simulink model "trasporto_impurezze"  (R2024b)
settings: Solver=VariableStepAuto  StartTime=0.0  StopTime=3  RelTol=1e-6
values from neighbouring files (symbols this model uses):
  ci_core = 2.05e19    (= 2.05e+19)    [fit_traporto_particelle.m]    (also in param_sparo_3.mat = 1.96393381569e+19)
  ci_omp = 1.0e19    (= 1e+19)    [fit_traporto_particelle.m]    (also in param_sparo_3.mat = 1.04458244578e+19)
  ci_T_core = 1071.06262207    [param_sparo_3.mat]
  ci_T_omp = 26.6552791595    [param_sparo_3.mat]
  ci_tar = 2.6e19    (= 2.6e+19)    [fit_traporto_particelle.m]    (also in param_sparo_3.mat = 1.50852693408e+19)
undefined symbols (not defined in the file or in its folder): ion, k0, Lz_valuesAzoto, V
libraries: slpidlib x3
settings Model: Creator=fedep  LastModifiedBy=costa

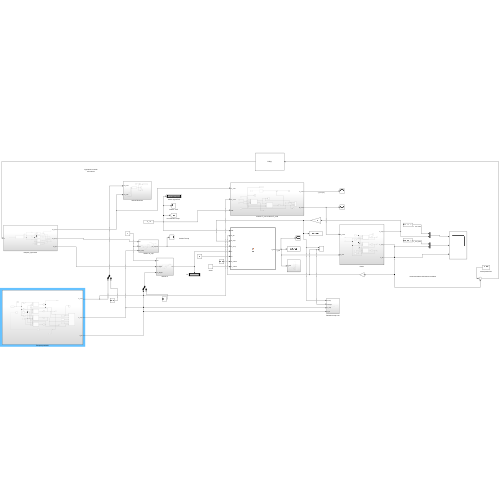
[thumbnail: Simulink's stored preview of the top-level diagram]
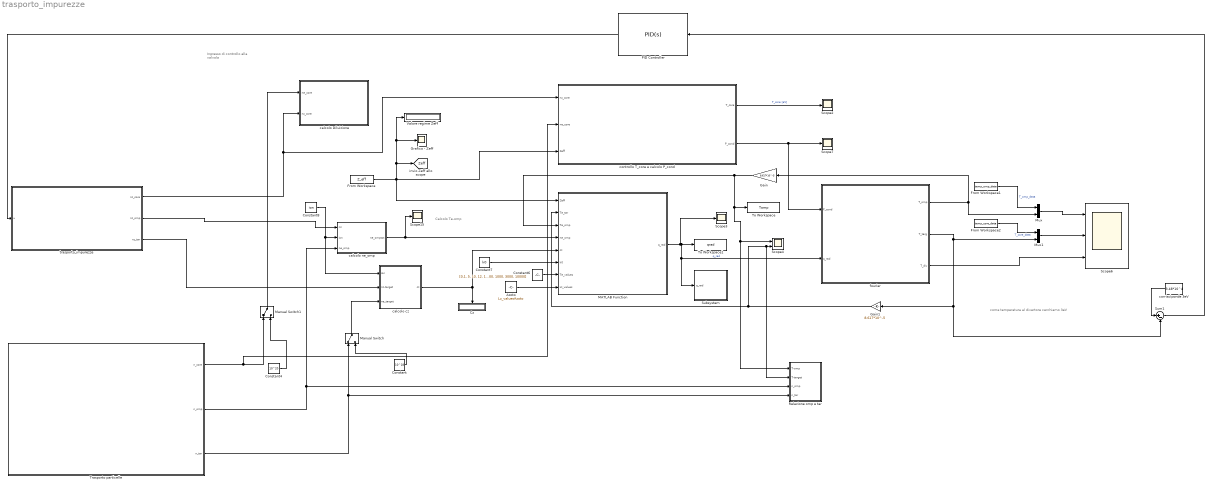
== system trasporto_impurezze ==
  note: come temperatura al divertore cerchiamo 3eV
  note: Ingresso di controllo
      | alla valvola
  note: Calcolo Te-omp
  Azoto : Constant  Value=Lz_valuesAzoto
  Constant : Constant  Value=10^18
  Constant4 : Constant  Value=10^20
  Constant6 : Constant  Value=[0,1, 5, 10, 12, 15, 20, 30, 59, 100, 155, 200, 300, 500, 700, 1000, 3000, 10000]
  Constant7 : Constant  Value=k0
  Constant8 : Constant  Value=ion
  Cz : Display
  From Workspace : FromWorkspace  VariableName=Z_eff
  From Workspace1 : FromWorkspace  VariableName=temp_omp_data
  From Workspace2 : FromWorkspace  VariableName=temp_core_data
  Gain : Gain  Gain=8.617*10^-5
  Gain1 : Gain  Gain=8.617*10^-5
  Grafico - Zeff : Scope
  MATLAB Function : MATLAB Function  TreatAsAtomicUnit=on
  Manual Switch : ManualSwitch
  Manual Switch1 : ManualSwitch
  Mux : Mux  Inputs=2
  Mux1 : Mux  Inputs=2
  PID Controller : slpidlib/PID Controller  Controller=PID  Form=Parallel  TimeDomain=Continuous-time  UseExternalTs=off  SampleTime=-1  IntegratorMethod=Forward Euler  FilterMethod=Forward Euler  ControllerParametersSource=internal  P=-7*10^9*0  I=-0.5*10^7*0  UseKiTs=off  D=-10^10*0  UseExternalDerivativeSource=off  N=100*0  UseFilter=on  TunerSelectOption=Transfer Function Based (PID Tuner App)  InitialConditionSource=internal  InitialConditionForIntegrator=0  InitialConditionForFilter=0  DifferentiatorICPrevScaledInput=0  ExternalReset=none  TrackingMode=off  Kt=1  LimitOutput=off  SatLimitsSource=internal  UpperSaturationLimit=inf  LowerSaturationLimit=-inf  LinearizeAsGain=on  AntiWindupMode=none  Kb=1  LimitIntegrator=off  UpperIntegratorSaturationLimit=inf  LowerIntegratorSaturationLimit=-inf  POutMin=[]  POutMax=[]  IOutMin=[]  IOutMax=[]  DOutMin=[]  DOutMax=[]  NOutMin=[]  NOutMax=[]  SumOutMin=[]  SumOutMax=[]  SaturationOutMin=[]  SaturationOutMax=[]  PParamMin=[]  PParamMax=[]  IParamMin=[]  IParamMax=[]  DParamMin=[]  DParamMax=[]  NParamMin=[]  NParamMax=[]  KbParamMin=[]  KbParamMax=[]  KtParamMin=[]  KtParamMax=[]  KbOutMin=[]  KbOutMax=[]  KtOutMin=[]  KtOutMax=[]  IntegratorOutMin=[]  IntegratorOutMax=[]  FilterOutMin=[]  FilterOutMax=[]  SumI1OutMin=[]  SumI1OutMax=[]  SumI2OutMin=[]  SumI2OutMax=[]  SumI3OutMin=[]  SumI3OutMax=[]  SumI4OutMin=[]  SumI4OutMax=[]  SumDOutMin=[]  SumDOutMax=[]  DifferentiatorOutMin=[]  DifferentiatorOutMax=[]  FilterDiffOutCoefMin=[]  FilterDiffOutCoefMax=[]  ReciprocalOutMin=[]  ReciprocalOutMax=[]  SumDenOutMin=[]  SumDenOutMax=[]  SumNumOutMin=[]  SumNumOutMax=[]  DivideOutMin=[]  DivideOutMax=[]  UdiffTsProdOutMin=[]  UdiffTsProdOutMax=[]  NTsProdOutMin=[]  NTsProdOutMax=[]  UintegralTsProdOutMin=[]  UintegralTsProdOutMax=[]  UngainTsProdOutMin=[]  UngainTsProdOutMax=[]  ClampingZeroOutDataTypeStr=Inherit: Inherit via back propagation  ClampingZeroOutMin=[]  ClampingZeroOutMax=[]  FilterDenConstantOutDataTypeStr=Inherit: Inherit via back propagation  FilterDenConstantOutMin=[]  FilterDenConstantOutMax=[]  PCopyOutDataTypeStr=Inherit: Inherit via back propagation  PCopyOutMin=[]  PCopyOutMax=[]  NCopyOutDataTypeStr=Inherit: Inherit via back propagation  NCopyOutMin=[]  NCopyOutMax=[]  IntegratorContinuousStateAttributes=''  IntegratorStateMustResolveToSignalObject=off  IntegratorRTWStateStorageClass=Auto  FilterContinuousStateAttributes=''  FilterStateMustResolveToSignalObject=off  FilterRTWStateStorageClass=Auto  ParallelPVariant=InternalParameters  IdealPVariant=Disabled  IVariant=InternalParameters  DVariant=InternalParameters  IntegratorVariant=Continuous  SatVariant=Disabled  AWVariant=Passthrough  PCopyVariant=Disabled  TRVariant=Disabled  FdbkBlocksVariant=Forward  IdealPFdbkVariant=Disabled  SatFdbkVariant=Disabled  DerivativeFilterVariant=ContFilter  NVariant=InternalParameters  NCopyVariant=Disabled  FilterICVariant=InternalICsFilter  IntegratorICVariant=InternalICs  ExternalResetVariant=Disabled  TRSumVariant=Passthrough  SumFdbkVariant=Disabled  SumVariant=Sum_PID  TsampFilterVariant=InternalTs  TsampNgainVariant=Passthrough  TsampIntegralVariant=Disabled_SignalSpec  ExternalSaturationOutDataTypeStr=Inherit: Same as second input  DerivativeSourceVariant=ErrorSignal  PreIntVariant=InternalPreInt
  Relazione omp e tar : Subsystem
  Scope{2..3,7,15} (4 alike) : Scope
  Scope4 : Scope  NumInputPorts=2
  Scope6 : Scope  NumInputPorts=3
  Subsystem : Subsystem
  Sum1 : Sum  Inputs=|+-
  To Workspace : ToWorkspace  VariableName=Tomp  SaveFormat=Timeseries  SampleTime=-1
  To Workspace1 : ToWorkspace  VariableName=qrad  SaveFormat=Timeseries  SampleTime=-1
  "Trasporto particelle " : Subsystem
  Valore regime Zeff : Display
  calcolo Diluizione : Subsystem
  calcolo cz : Subsystem
  calcolo ne_omp : Subsystem
  controllo T_core e calcolo P_cond : Subsystem
  corriscìponde 3eV : Constant  Value=3.48*10^4
  fourier : Subsystem
  trasporto_impurezze : Subsystem
  tag scope: Zeff=global
  wires:
  Constant6/1 -> MATLAB Function/7(Te_values)
  "Trasporto particelle "/1(n_core) -> controllo T_core e calcolo P_cond/2(ne_core), Manual Switch1/1
  "Trasporto particelle "/3(n_tar) -> Manual Switch/1, Relazione omp e tar/4(n_tar)
  Azoto/1 -> MATLAB Function/8(Lz_values)
  Manual Switch/1 -> calcolo cz/3(ne_target)
  Constant8/1 -> calcolo cz/1(ion), calcolo ne_omp/2(ion)
  From Workspace/1 -> controllo T_core e calcolo P_cond/3(Zeff), [Zeff], Grafico - Zeff/1, Valore regime Zeff/1, MATLAB Function/1(Zeff)
  Manual Switch1/1 -> calcolo Diluizione/1(ne_core)
  MATLAB Function/1(q_rad) -> To Workspace1/1, fourier/2(q_rad), Subsystem/1(q_rad), Scope3/1  "q_rad"
  "Trasporto particelle "/2(n_omp) -> calcolo ne_omp/3(ne_omp), Relazione omp e tar/3(n_omp)
  fourier/1(T_omp) -> Mux/2, Gain/1
  trasporto_impurezze/2(nz_omp) -> calcolo ne_omp/1(nz)
  PID Controller/1 -> trasporto_impurezze/1(u)
  fourier/3(T_div) -> Scope6/3
  Constant4/1 -> Manual Switch1/2
  corriscìponde 3eV/1 -> Sum1/1
  Sum1/1 -> PID Controller/1
  controllo T_core e calcolo P_cond/1(T_core) -> Scope2/1  "T_core [eV]"
  controllo T_core e calcolo P_cond/2(P_cond) -> Scope7/1, fourier/1(P_cond)
  calcolo ne_omp/1(ne_omptot) -> MATLAB Function/4(ne_omp), Scope15/1
  Gain/1 -> To Workspace/1, Relazione omp e tar/1(T-omp), Scope4/1, MATLAB Function/3(Te_omp)
  Constant/1 -> Manual Switch/2
  Constant7/1 -> MATLAB Function/6(k0)
  fourier/2(T_targ) -> Sum1/2, Gain1/1, Mux1/2
  Gain1/1 -> Scope4/2, Relazione omp e tar/2(T-target), MATLAB Function/2(Te_tar)
  calcolo cz/1(cz) -> Cz/1, MATLAB Function/5(cz)
  trasporto_impurezze/1(nz_core) -> calcolo Diluizione/2(nz_core), controllo T_core e calcolo P_cond/1(nz_core)
  trasporto_impurezze/3(nz_tar) -> calcolo cz/2(nz-target)
  From Workspace1/1 -> Mux/1  "T_omp_data"
  From Workspace2/1 -> Mux1/1  "T_core_data"
  Mux/1 -> Scope6/1
  Mux1/1 -> Scope6/2

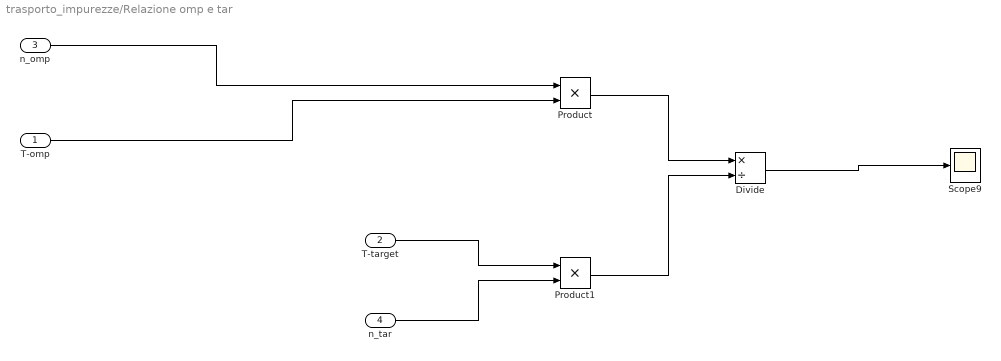
== system trasporto_impurezze/Relazione omp e tar ==
  T-omp : Inport
  T-target : Inport  Port=2
  n_omp : Inport  Port=3
  n_tar : Inport  Port=4
  Divide : Product  Inputs=*/
  Product : Product
  Product1 : Product
  Scope9 : Scope
  wires:
  Product/1 -> Divide/1
  n_tar/1 -> Product1/2
  Divide/1 -> Scope9/1
  Product1/1 -> Divide/2
  n_omp/1 -> Product/1
  T-target/1 -> Product1/1
  T-omp/1 -> Product/2

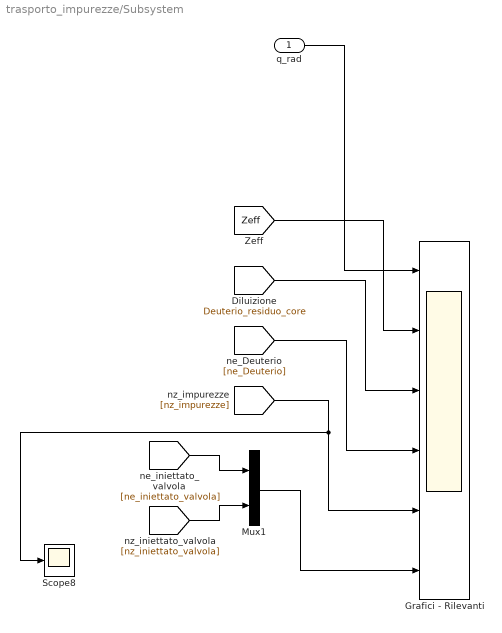
== system trasporto_impurezze/Subsystem ==
  q_rad : Inport
  Grafici - Rilevanti : Scope  NumInputPorts=6
  Mux1 : Mux  Inputs=2
  Scope8 : Scope
  wires:
  q_rad/1 -> Grafici - Rilevanti/1
  [Zeff] -> Grafici - Rilevanti/2
  [nz_impurezze] -> Scope8/1, Grafici - Rilevanti/5
  Mux1/1 -> Grafici - Rilevanti/6
  [nz_iniettato_valvola] -> Mux1/2
  [Deuterio_residuo_core] -> Grafici - Rilevanti/3
  [ne_Deuterio] -> Grafici - Rilevanti/4
  [ne_iniettato_valvola] -> Mux1/1

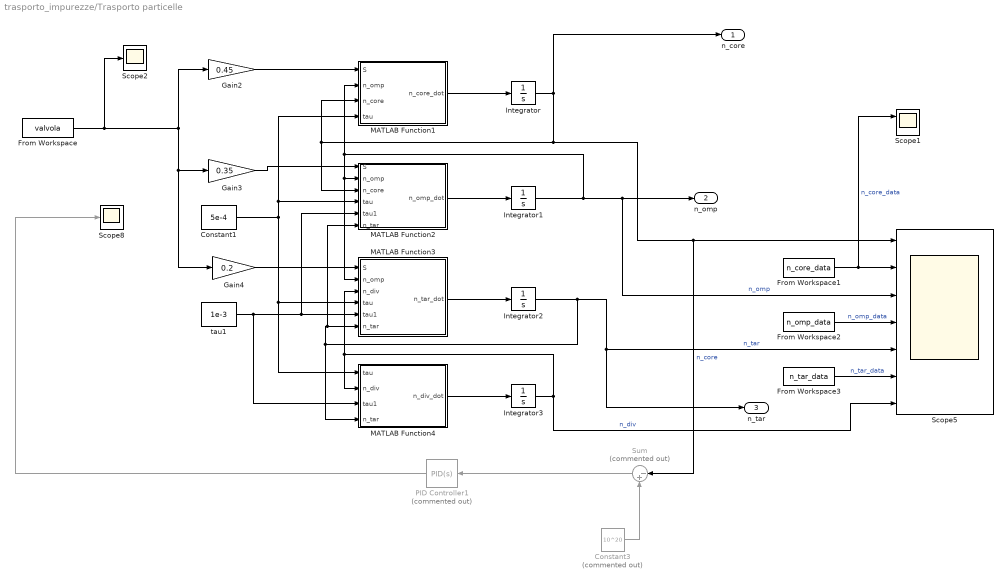
== system trasporto_impurezze/Trasporto particelle  ==
  Constant1 : Constant  Value=5e-4
  Constant3 : Constant  Commented=on  Value=10^20
  From Workspace : FromWorkspace  VariableName=valvola
  From Workspace1 : FromWorkspace  VariableName=n_core_data
  From Workspace2 : FromWorkspace  VariableName=n_omp_data
  From Workspace3 : FromWorkspace  VariableName=n_tar_data
  Gain2 : Gain  Gain=0.45
  Gain3 : Gain  Gain=0.35
  Gain4 : Gain  Gain=0.2
  Integrator : Integrator  InitialCondition=ci_core
  Integrator1 : Integrator  InitialCondition=ci_omp
  Integrator2 : Integrator  InitialCondition=ci_tar
  Integrator3 : Integrator  InitialCondition=10^10
  MATLAB Function1 : MATLAB Function  TreatAsAtomicUnit=on
  MATLAB Function2 : MATLAB Function  TreatAsAtomicUnit=on
  MATLAB Function3 : MATLAB Function  TreatAsAtomicUnit=on
  MATLAB Function4 : MATLAB Function  TreatAsAtomicUnit=on
  PID Controller1 : slpidlib/PID Controller  Commented=on  Controller=PID  Form=Parallel  TimeDomain=Continuous-time  UseExternalTs=off  SampleTime=-1  IntegratorMethod=Forward Euler  FilterMethod=Forward Euler  ControllerParametersSource=internal  P=10^2  I=0  UseKiTs=off  D=0  UseExternalDerivativeSource=off  N=100  UseFilter=on  TunerSelectOption=Transfer Function Based (PID Tuner App)  InitialConditionSource=internal  InitialConditionForIntegrator=0  InitialConditionForFilter=0  DifferentiatorICPrevScaledInput=0  ExternalReset=none  TrackingMode=off  Kt=1  LimitOutput=off  SatLimitsSource=internal  UpperSaturationLimit=inf  LowerSaturationLimit=-inf  LinearizeAsGain=on  AntiWindupMode=none  Kb=1  LimitIntegrator=off  UpperIntegratorSaturationLimit=inf  LowerIntegratorSaturationLimit=-inf  POutMin=[]  POutMax=[]  IOutMin=[]  IOutMax=[]  DOutMin=[]  DOutMax=[]  NOutMin=[]  NOutMax=[]  SumOutMin=[]  SumOutMax=[]  SaturationOutMin=[]  SaturationOutMax=[]  PParamMin=[]  PParamMax=[]  IParamMin=[]  IParamMax=[]  DParamMin=[]  DParamMax=[]  NParamMin=[]  NParamMax=[]  KbParamMin=[]  KbParamMax=[]  KtParamMin=[]  KtParamMax=[]  KbOutMin=[]  KbOutMax=[]  KtOutMin=[]  KtOutMax=[]  IntegratorOutMin=[]  IntegratorOutMax=[]  FilterOutMin=[]  FilterOutMax=[]  SumI1OutMin=[]  SumI1OutMax=[]  SumI2OutMin=[]  SumI2OutMax=[]  SumI3OutMin=[]  SumI3OutMax=[]  SumI4OutMin=[]  SumI4OutMax=[]  SumDOutMin=[]  SumDOutMax=[]  DifferentiatorOutMin=[]  DifferentiatorOutMax=[]  FilterDiffOutCoefMin=[]  FilterDiffOutCoefMax=[]  ReciprocalOutMin=[]  ReciprocalOutMax=[]  SumDenOutMin=[]  SumDenOutMax=[]  SumNumOutMin=[]  SumNumOutMax=[]  DivideOutMin=[]  DivideOutMax=[]  UdiffTsProdOutMin=[]  UdiffTsProdOutMax=[]  NTsProdOutMin=[]  NTsProdOutMax=[]  UintegralTsProdOutMin=[]  UintegralTsProdOutMax=[]  UngainTsProdOutMin=[]  UngainTsProdOutMax=[]  ClampingZeroOutDataTypeStr=Inherit: Inherit via back propagation  ClampingZeroOutMin=[]  ClampingZeroOutMax=[]  FilterDenConstantOutDataTypeStr=Inherit: Inherit via back propagation  FilterDenConstantOutMin=[]  FilterDenConstantOutMax=[]  PCopyOutDataTypeStr=Inherit: Inherit via back propagation  PCopyOutMin=[]  PCopyOutMax=[]  NCopyOutDataTypeStr=Inherit: Inherit via back propagation  NCopyOutMin=[]  NCopyOutMax=[]  IntegratorContinuousStateAttributes=''  IntegratorStateMustResolveToSignalObject=off  IntegratorRTWStateStorageClass=Auto  FilterContinuousStateAttributes=''  FilterStateMustResolveToSignalObject=off  FilterRTWStateStorageClass=Auto  ParallelPVariant=InternalParameters  IdealPVariant=Disabled  IVariant=InternalParameters  DVariant=InternalParameters  IntegratorVariant=Continuous  SatVariant=Disabled  AWVariant=Passthrough  PCopyVariant=Disabled  TRVariant=Disabled  FdbkBlocksVariant=Forward  IdealPFdbkVariant=Disabled  SatFdbkVariant=Disabled  DerivativeFilterVariant=ContFilter  NVariant=InternalParameters  NCopyVariant=Disabled  FilterICVariant=InternalICsFilter  IntegratorICVariant=InternalICs  ExternalResetVariant=Disabled  TRSumVariant=Passthrough  SumFdbkVariant=Disabled  SumVariant=Sum_PID  TsampFilterVariant=InternalTs  TsampNgainVariant=Passthrough  TsampIntegralVariant=Disabled_SignalSpec  ExternalSaturationOutDataTypeStr=Inherit: Same as second input  DerivativeSourceVariant=ErrorSignal  PreIntVariant=InternalPreInt
  Scope1 : Scope  NumInputPorts=2
  Scope2 : Scope
  Scope5 : Scope  NumInputPorts=7
  Scope8 : Scope
  Sum : Sum  Commented=on  Inputs=|-+
  tau1 : Constant  Value=1e-3
  n_core : Outport
  n_omp : Outport  Port=2
  n_tar : Outport  Port=3
  wires:
  Gain3/1 -> MATLAB Function2/1(S)
  Integrator2/1 -> n_tar/1, Scope5/5, MATLAB Function4/4(n_tar), MATLAB Function2/6(n_tar), MATLAB Function3/6(n_tar)  "n_tar"
  MATLAB Function2/1(n_omp_dot) -> Integrator1/1
  Integrator/1 -> n_core/1, Sum/1, Scope5/1, MATLAB Function1/3(n_core), MATLAB Function2/3(n_core)  "n_core"
  Integrator1/1 -> MATLAB Function3/2(n_omp), MATLAB Function2/2(n_omp), MATLAB Function1/2(n_omp), Scope5/3, n_omp/1  "n_omp"
  Constant1/1 -> MATLAB Function1/4(tau), MATLAB Function2/4(tau), MATLAB Function4/1(tau), MATLAB Function3/4(tau)
  Gain4/1 -> MATLAB Function3/1(S)
  Gain2/1 -> MATLAB Function1/1(S)
  MATLAB Function1/1(n_core_dot) -> Integrator/1
  Integrator3/1 -> MATLAB Function4/2(n_div), MATLAB Function3/3(n_div), Scope5/7  "n_div"
  MATLAB Function4/1(n_div_dot) -> Integrator3/1
  MATLAB Function3/1(n_tar_dot) -> Integrator2/1
  Sum/1 -> PID Controller1/1
  Constant3/1 -> Sum/2
  PID Controller1/1 -> Scope8/1
  From Workspace/1 -> Scope2/1, Gain2/1, Gain4/1, Gain3/1
  From Workspace1/1 -> Scope1/1, Scope5/2  "n_core_data"
  From Workspace2/1 -> Scope5/4  "n_omp_data"
  From Workspace3/1 -> Scope5/6  "n_tar_data"
  tau1/1 -> MATLAB Function4/3(tau1), MATLAB Function2/5(tau1), MATLAB Function3/5(tau1)

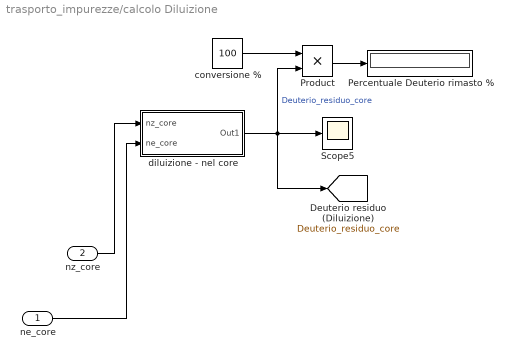
== system trasporto_impurezze/calcolo Diluizione ==
  ne_core : Inport
  nz_core : Inport  Port=2
  Percentuale Deuterio rimasto % : Display
  Product : Product
  Scope5 : Scope
  "conversione % " : Constant  Value=100
  diluizione - nel core : Subsystem
  tag scope: Deuterio_residuo_core=global
  wires:
  Product/1 -> Percentuale Deuterio rimasto %/1
  nz_core/1 -> diluizione - nel core/1(nz_core)
  "conversione % "/1 -> Product/1
  diluizione - nel core/1(Out1) -> [Deuterio_residuo_core], Scope5/1, Product/2  "Deuterio_residuo_core"
  ne_core/1 -> diluizione - nel core/2(ne_core)

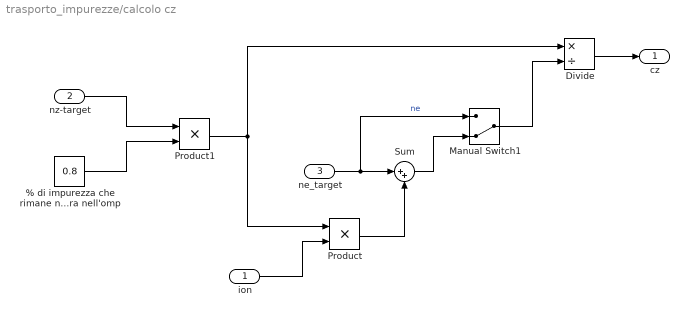
== system trasporto_impurezze/calcolo cz ==
  ion : Inport
  nz-target : Inport  Port=2
  ne_target : Inport  Port=3
  % di impurezza che rimane nel div. Parte restante migra nell'omp : Constant  Value=0.8
  Divide : Product  Inputs=*/
  Manual Switch1 : ManualSwitch  CurrentSetting=0
  Product : Product
  Product1 : Product
  Sum : Sum  Inputs=|++
  cz : Outport
  wires:
  ne_target/1 -> Manual Switch1/1, Sum/1  "ne"
  Sum/1 -> Manual Switch1/2
  Divide/1 -> cz/1
  Manual Switch1/1 -> Divide/2
  Product/1 -> Sum/2
  nz-target/1 -> Product1/1
  % di impurezza che rimane nel div. Parte restante migra nell'omp/1 -> Product1/2
  ion/1 -> Product/2
  Product1/1 -> Divide/1, Product/1

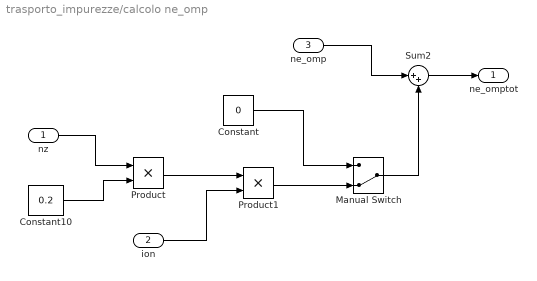
== system trasporto_impurezze/calcolo ne_omp ==
  nz : Inport
  ion : Inport  Port=2
  ne_omp : Inport  Port=3
  Constant : Constant  Value=0
  Constant10 : Constant  Value=0.2
  Manual Switch : ManualSwitch  CurrentSetting=0
  Product : Product
  Product1 : Product
  Sum2 : Sum  Inputs=|++
  ne_omptot : Outport
  wires:
  Constant10/1 -> Product/2
  Sum2/1 -> ne_omptot/1
  nz/1 -> Product/1
  ne_omp/1 -> Sum2/1
  Constant/1 -> Manual Switch/1
  Manual Switch/1 -> Sum2/2
  Product/1 -> Product1/1
  ion/1 -> Product1/2
  Product1/1 -> Manual Switch/2

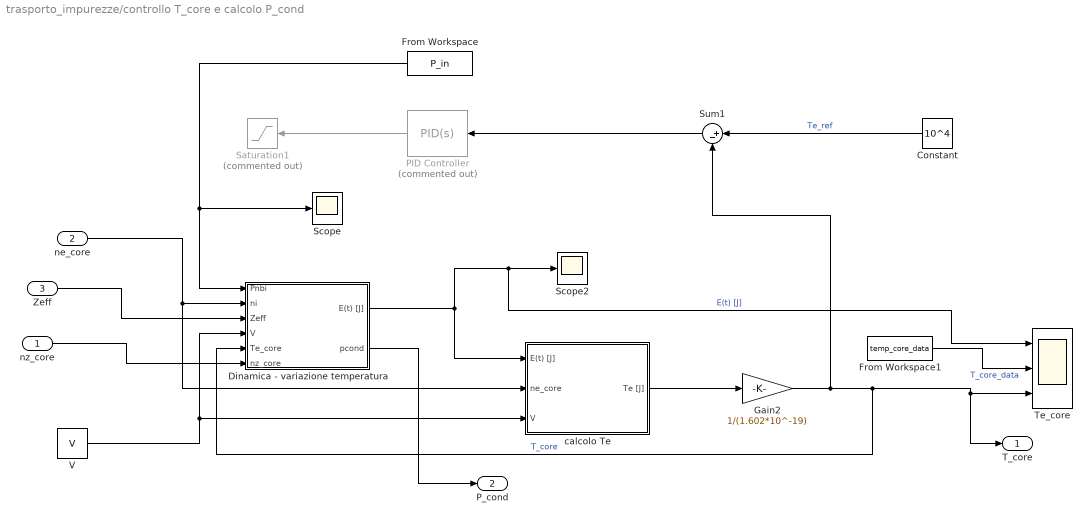
== system trasporto_impurezze/controllo T_core e calcolo P_cond ==
  nz_core : Inport
  ne_core : Inport  Port=2
  Zeff : Inport  Port=3
  Constant : Constant  Value=10^4
  Dinamica - variazione temperatura : Subsystem
  From Workspace : FromWorkspace  VariableName=P_in
  From Workspace1 : FromWorkspace  VariableName=temp_core_data
  Gain2 : Gain  Gain=1/(1.602*10^-19)
  PID Controller : slpidlib/PID Controller  Commented=on  Controller=PID  Form=Parallel  TimeDomain=Continuous-time  UseExternalTs=off  SampleTime=-1  IntegratorMethod=Forward Euler  FilterMethod=Forward Euler  ControllerParametersSource=internal  P=18958.3832510532  I=195534.723934352  UseKiTs=off  D=-5.96212634512888  UseExternalDerivativeSource=off  N=3179.8023311838  UseFilter=on  TunerSelectOption=Transfer Function Based (PID Tuner App)  InitialConditionSource=internal  InitialConditionForIntegrator=0  InitialConditionForFilter=0  DifferentiatorICPrevScaledInput=0  ExternalReset=none  TrackingMode=off  Kt=1  LimitOutput=off  SatLimitsSource=internal  UpperSaturationLimit=inf  LowerSaturationLimit=-inf  LinearizeAsGain=on  AntiWindupMode=none  Kb=1  LimitIntegrator=off  UpperIntegratorSaturationLimit=inf  LowerIntegratorSaturationLimit=-inf  POutMin=[]  POutMax=[]  IOutMin=[]  IOutMax=[]  DOutMin=[]  DOutMax=[]  NOutMin=[]  NOutMax=[]  SumOutMin=[]  SumOutMax=[]  SaturationOutMin=[]  SaturationOutMax=[]  PParamMin=[]  PParamMax=[]  IParamMin=[]  IParamMax=[]  DParamMin=[]  DParamMax=[]  NParamMin=[]  NParamMax=[]  KbParamMin=[]  KbParamMax=[]  KtParamMin=[]  KtParamMax=[]  KbOutMin=[]  KbOutMax=[]  KtOutMin=[]  KtOutMax=[]  IntegratorOutMin=[]  IntegratorOutMax=[]  FilterOutMin=[]  FilterOutMax=[]  SumI1OutMin=[]  SumI1OutMax=[]  SumI2OutMin=[]  SumI2OutMax=[]  SumI3OutMin=[]  SumI3OutMax=[]  SumI4OutMin=[]  SumI4OutMax=[]  SumDOutMin=[]  SumDOutMax=[]  DifferentiatorOutMin=[]  DifferentiatorOutMax=[]  FilterDiffOutCoefMin=[]  FilterDiffOutCoefMax=[]  ReciprocalOutMin=[]  ReciprocalOutMax=[]  SumDenOutMin=[]  SumDenOutMax=[]  SumNumOutMin=[]  SumNumOutMax=[]  DivideOutMin=[]  DivideOutMax=[]  UdiffTsProdOutMin=[]  UdiffTsProdOutMax=[]  NTsProdOutMin=[]  NTsProdOutMax=[]  UintegralTsProdOutMin=[]  UintegralTsProdOutMax=[]  UngainTsProdOutMin=[]  UngainTsProdOutMax=[]  ClampingZeroOutDataTypeStr=Inherit: Inherit via back propagation  ClampingZeroOutMin=[]  ClampingZeroOutMax=[]  FilterDenConstantOutDataTypeStr=Inherit: Inherit via back propagation  FilterDenConstantOutMin=[]  FilterDenConstantOutMax=[]  PCopyOutDataTypeStr=Inherit: Inherit via back propagation  PCopyOutMin=[]  PCopyOutMax=[]  NCopyOutDataTypeStr=Inherit: Inherit via back propagation  NCopyOutMin=[]  NCopyOutMax=[]  IntegratorContinuousStateAttributes=''  IntegratorStateMustResolveToSignalObject=off  IntegratorRTWStateStorageClass=Auto  FilterContinuousStateAttributes=''  FilterStateMustResolveToSignalObject=off  FilterRTWStateStorageClass=Auto  ParallelPVariant=InternalParameters  IdealPVariant=Disabled  IVariant=InternalParameters  DVariant=InternalParameters  IntegratorVariant=Continuous  SatVariant=Disabled  AWVariant=Passthrough  PCopyVariant=Disabled  TRVariant=Disabled  FdbkBlocksVariant=Forward  IdealPFdbkVariant=Disabled  SatFdbkVariant=Disabled  DerivativeFilterVariant=ContFilter  NVariant=InternalParameters  NCopyVariant=Disabled  FilterICVariant=InternalICsFilter  IntegratorICVariant=InternalICs  ExternalResetVariant=Disabled  TRSumVariant=Passthrough  SumFdbkVariant=Disabled  SumVariant=Sum_PID  TsampFilterVariant=InternalTs  TsampNgainVariant=Passthrough  TsampIntegralVariant=Disabled_SignalSpec  ExternalSaturationOutDataTypeStr=Inherit: Same as second input  DerivativeSourceVariant=ErrorSignal  PreIntVariant=InternalPreInt
  Saturation1 : Saturate  Commented=on  UpperLimit=inf  LowerLimit=0
  Scope : Scope
  Scope2 : Scope
  Sum1 : Sum  Inputs=|+-
  Te_core : Scope  NumInputPorts=3
  V : Constant  Value=V
  calcolo Te : Subsystem
  T_core : Outport
  P_cond : Outport  Port=2
  wires:
  Constant/1 -> Sum1/1  "Te_ref"
  Gain2/1 -> Sum1/2, Dinamica - variazione temperatura/5(Te_core), Te_core/3, T_core/1  "T_core"
  Zeff/1 -> Dinamica - variazione temperatura/3(Zeff)
  ne_core/1 -> calcolo Te/2(ne_core), Dinamica - variazione temperatura/2(ni)
  V/1 -> calcolo Te/3(V), Dinamica - variazione temperatura/4(V)
  PID Controller/1 -> Saturation1/1
  Dinamica - variazione temperatura/1(E(t) [J]) -> Te_core/1, Scope2/1, calcolo Te/1(E(t) [J])  "E(t) [J]"
  Sum1/1 -> PID Controller/1
  nz_core/1 -> Dinamica - variazione temperatura/6(nz_core)
  Dinamica - variazione temperatura/2(pcond) -> P_cond/1
  calcolo Te/1(Te [J]) -> Gain2/1
  From Workspace/1 -> Scope/1, Dinamica - variazione temperatura/1(Pnbi)
  From Workspace1/1 -> Te_core/2  "T_core_data"

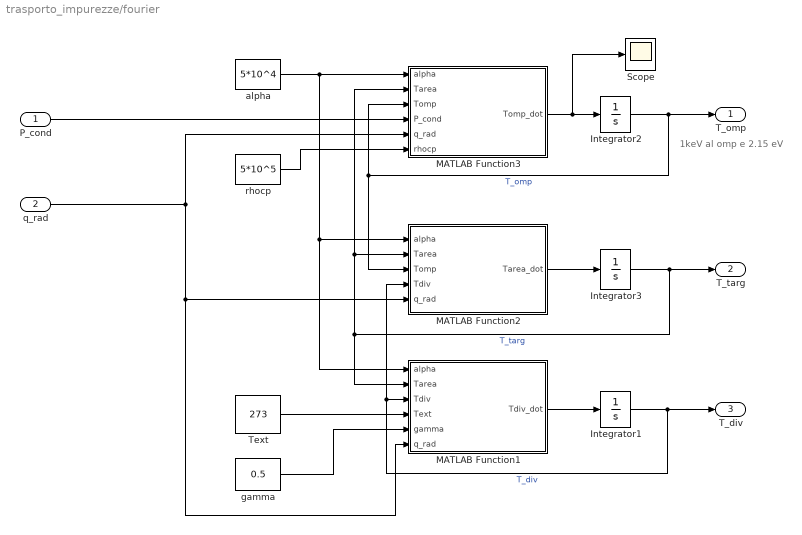
== system trasporto_impurezze/fourier ==
  note: 1keV al omp e 2.15 eV
  P_cond : Inport
  q_rad : Inport  Port=2
  Integrator1 : Integrator  InitialCondition=275
  Integrator2 : Integrator  InitialCondition=ci_T_omp
  Integrator3 : Integrator  InitialCondition=ci_T_core
  MATLAB Function1 : MATLAB Function  TreatAsAtomicUnit=on
  MATLAB Function2 : MATLAB Function  TreatAsAtomicUnit=on
  MATLAB Function3 : MATLAB Function  TreatAsAtomicUnit=on
  Scope : Scope
  Text : Constant  Value=273
  alpha : Constant  Value=5*10^4
  gamma : Constant  Value=0.5
  rhocp : Constant  Value=5*10^5
  T_omp : Outport
  T_targ : Outport  Port=2
  T_div : Outport  Port=3
  wires:
  alpha/1 -> MATLAB Function1/1(alpha), MATLAB Function2/1(alpha), MATLAB Function3/1(alpha)
  MATLAB Function3/1(Tomp_dot) -> Scope/1, Integrator2/1
  Text/1 -> MATLAB Function1/4(Text)
  Integrator1/1 -> T_div/1, MATLAB Function2/4(Tdiv), MATLAB Function1/3(Tdiv)  "T_div"
  P_cond/1 -> MATLAB Function3/4(P_cond)
  q_rad/1 -> MATLAB Function3/5(q_rad), MATLAB Function2/5(q_rad), MATLAB Function1/6(q_rad)
  gamma/1 -> MATLAB Function1/5(gamma)
  MATLAB Function2/1(Tarea_dot) -> Integrator3/1
  MATLAB Function1/1(Tdiv_dot) -> Integrator1/1
  Integrator2/1 -> T_omp/1, MATLAB Function3/3(Tomp), MATLAB Function2/3(Tomp)  "T_omp"
  Integrator3/1 -> MATLAB Function3/2(Tarea), MATLAB Function2/2(Tarea), MATLAB Function1/2(Tarea), T_targ/1  "T_targ"
  rhocp/1 -> MATLAB Function3/6(rhocp)

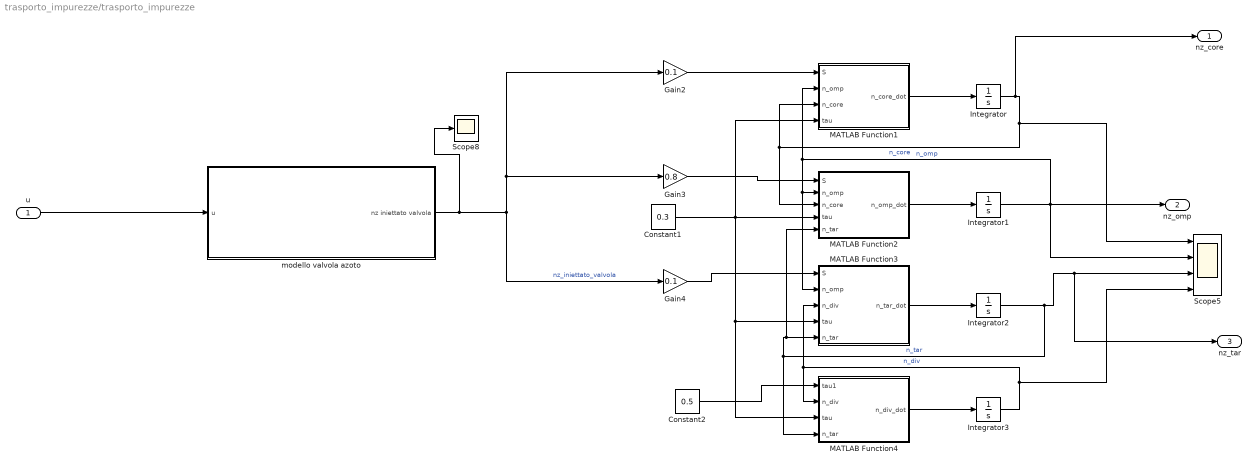
== system trasporto_impurezze/trasporto_impurezze ==
  u : Inport
  Constant1 : Constant  Value=0.3
  Constant2 : Constant  Value=0.5
  Gain2 : Gain  Gain=0.1
  Gain3 : Gain  Gain=0.8
  Gain4 : Gain  Gain=0.1
  Integrator{,1..3} (4 alike) : Integrator
  MATLAB Function1 : MATLAB Function  TreatAsAtomicUnit=on
  MATLAB Function2 : MATLAB Function  TreatAsAtomicUnit=on
  MATLAB Function3 : MATLAB Function  TreatAsAtomicUnit=on
  MATLAB Function4 : MATLAB Function  TreatAsAtomicUnit=on
  Scope5 : Scope  NumInputPorts=4
  Scope8 : Scope
  modello valvola azoto : Subsystem
  nz_core : Outport
  nz_omp : Outport  Port=2
  nz_tar : Outport  Port=3
  wires:
  u/1 -> modello valvola azoto/1(u)
  Integrator/1 -> nz_core/1, Scope5/1, MATLAB Function1/3(n_core), MATLAB Function2/3(n_core)  "n_core"
  MATLAB Function1/1(n_core_dot) -> Integrator/1
  Constant2/1 -> MATLAB Function4/1(tau1)
  Constant1/1 -> MATLAB Function1/4(tau), MATLAB Function2/4(tau), MATLAB Function4/3(tau), MATLAB Function3/4(tau)
  Integrator1/1 -> nz_omp/1, Scope5/2, MATLAB Function3/2(n_omp), MATLAB Function2/2(n_omp), MATLAB Function1/2(n_omp)  "n_omp"
  Integrator3/1 -> Scope5/4, MATLAB Function4/2(n_div), MATLAB Function3/3(n_div)  "n_div"
  Gain3/1 -> MATLAB Function2/1(S)
  MATLAB Function3/1(n_tar_dot) -> Integrator2/1
  Gain2/1 -> MATLAB Function1/1(S)
  MATLAB Function4/1(n_div_dot) -> Integrator3/1
  MATLAB Function2/1(n_omp_dot) -> Integrator1/1
  Gain4/1 -> MATLAB Function3/1(S)
  Integrator2/1 -> MATLAB Function4/4(n_tar), MATLAB Function2/5(n_tar), MATLAB Function3/5(n_tar), nz_tar/1, Scope5/3  "n_tar"
  modello valvola azoto/1(nz iniettato valvola) -> Scope8/1, Gain3/1, Gain2/1, Gain4/1  "nz_iniettato_valvola"

== system trasporto_impurezze/calcolo Diluizione/diluizione - nel core ==
  nz_core : Inport
  ne_core : Inport  Port=2
  Divide : Product  Inputs=/*
  Product : Product
  Subtract : Sum  Inputs=+-
  Tasso di ionizzazione : Constant  Value=ion
  Out1 : Outport
  wires:
  nz_core/1 -> Product/1
  Tasso di ionizzazione/1 -> Product/2
  ne_core/1 -> Subtract/1, Divide/1
  Product/1 -> Subtract/2
  Divide/1 -> Out1/1
  Subtract/1 -> Divide/2

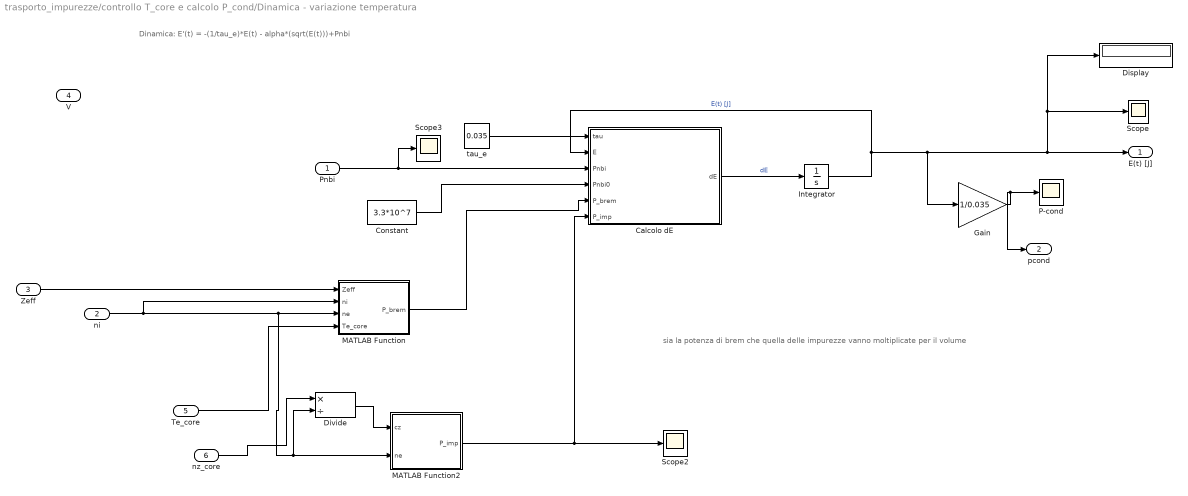
== system trasporto_impurezze/controllo T_core e calcolo P_cond/Dinamica - variazione temperatura ==
  note: sia la potenza di brem che quella delle impurezze vanno moltiplicate per il volume
  note: Dinamica: E'(t) = -(1/tau_e)*E(t) - alpha*(sqrt(E(t)))+Pnbi
  Pnbi : Inport
  ni : Inport  Port=2
  Zeff : Inport  Port=3
  V : Inport  Port=4
  Te_core : Inport  Port=5
  nz_core : Inport  Port=6
  Calcolo dE : MATLAB Function  TreatAsAtomicUnit=on
  Constant : Constant  Value=3.3*10^7
  Display : Display
  Divide : Product  Inputs=*/
  Gain : Gain  Gain=1/0.035
  Integrator : Integrator
  MATLAB Function : MATLAB Function  TreatAsAtomicUnit=on
  MATLAB Function2 : MATLAB Function  TreatAsAtomicUnit=on
  P-cond : Scope
  Scope : Scope
  Scope2 : Scope
  Scope3 : Scope
  tau_e : Constant  Value=0.035
  E(t) [J] : Outport
  pcond : Outport  Port=2
  wires:
  Calcolo dE/1(dE) -> Integrator/1  "dE"
  tau_e/1 -> Calcolo dE/1(tau)
  ni/1 -> MATLAB Function/2(ni), MATLAB Function2/2(ne), Divide/2, MATLAB Function/3(ne)
  Zeff/1 -> MATLAB Function/1(Zeff)
  Pnbi/1 -> Scope3/1, Calcolo dE/3(Pnbi)
  Gain/1 -> pcond/1, P-cond/1
  Constant/1 -> Calcolo dE/4(Pnbi0)
  Integrator/1 -> Calcolo dE/2(E), Gain/1, Display/1, Scope/1, E(t) [J]/1  "E(t) [J]"
  MATLAB Function/1(P_brem) -> Calcolo dE/5(P_brem)
  Te_core/1 -> MATLAB Function/4(Te_core)
  nz_core/1 -> Divide/1
  Divide/1 -> MATLAB Function2/1(cz)
  MATLAB Function2/1(P_imp) -> Scope2/1, Calcolo dE/6(P_imp)

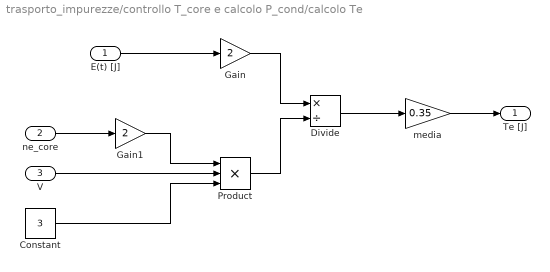
== system trasporto_impurezze/controllo T_core e calcolo P_cond/calcolo Te ==
  E(t) [J] : Inport
  ne_core : Inport  Port=2
  V : Inport  Port=3
  Constant : Constant  Value=3
  Divide : Product  Inputs=*/
  Gain : Gain  Gain=2
  Gain1 : Gain  Gain=2
  Product : Product  Inputs=3
  media : Gain  Gain=0.35
  Te [J] : Outport
  wires:
  ne_core/1 -> Gain1/1
  V/1 -> Product/2
  Constant/1 -> Product/3
  E(t) [J]/1 -> Gain/1
  Gain/1 -> Divide/1
  Product/1 -> Divide/2
  Divide/1 -> media/1
  Gain1/1 -> Product/1
  media/1 -> Te [J]/1

== system trasporto_impurezze/trasporto_impurezze/modello valvola azoto ==
  u : Inport
  Saturation : Saturate  UpperLimit=inf  LowerLimit=0
  Transfer Fcn : TransferFcn  Numerator=[0.91]  Denominator=[0.002 1]
  Transport Delay : TransportDelay  DelayTime=0.0019
  nz iniettato valvola : Outport
  wires:
  Transfer Fcn/1 -> Saturation/1  "nz"
  Transport Delay/1 -> Transfer Fcn/1
  u/1 -> Transport Delay/1
  Saturation/1 -> nz iniettato valvola/1

== matlab function trasporto_impurezze/MATLAB Function2 ==
  data: S input; n_omp_dot output; n_omp input; n_core input; tau input; n_tar input
function n_omp_dot = fcn(S, n_omp,n_core,tau, n_tar)
    n_omp_dot =  S+(n_core-n_omp)/tau+(n_omp-n_tar)/0.2 ;
    n_omp_dot = 0;
end

== matlab function trasporto_impurezze/MATLAB Function3 ==
  data: S input; n_tar_dot output; n_omp input; n_div input; tau input; n_tar input
function n_tar_dot = fcn(S, n_omp,n_div,tau, n_tar)
    n_tar_dot =  S+(n_omp-n_tar)/0.2+(n_tar-n_div)/tau;
    n_tar_dot = 0;
end

== matlab function trasporto_impurezze/MATLAB Function4 ==
  data: tau1 input; n_div_dot output; n_div input; tau input; n_tar input
function n_div_dot = fcn(tau1,n_div,tau, n_tar)
    n_div_dot =  (n_tar-n_div)/tau-(n_div)/tau1;
    n_div_dot = 0;
end

== matlab function trasporto_impurezze/Trasporto particelle /MATLAB Function1 ==
  data: S input; n_core_dot output; n_omp input; n_core input; tau input
function n_core_dot = fcn(S, n_omp,n_core,tau)
    n_core_dot =  S+(n_omp-n_core)/tau;
    % tau è il denominatore
end

== matlab function trasporto_impurezze/Trasporto particelle /MATLAB Function2 ==
  data: S input; n_omp_dot output; n_omp input; n_core input; tau input; tau1 input; n_tar input
function n_omp_dot = fcn(S, n_omp, n_core, tau, tau1, n_tar)
    % tau = 200;
    n_omp_dot =  S+(n_core-n_omp)/tau+(n_tar-n_omp)/tau1 ;
    %n_omp_dot =  S+(n_tar-n_omp)/8 ;
end

== matlab function trasporto_impurezze/Trasporto particelle /MATLAB Function3 ==
  data: S input; n_tar_dot output; n_omp input; n_div input; tau input; tau1 input; n_tar input
function n_tar_dot = fcn(S, n_omp, n_div, tau, tau1, n_tar)
    % tau1 = 0.005;
    % tau = 0.0002;
    n_tar_dot =  S+(n_omp-n_tar)/tau+(n_div-n_tar)/tau;
end

== matlab function trasporto_impurezze/MATLAB Function ==
  data: q_rad output; Zeff input; Te_tar input; Te_omp input; ne_omp input; cz input; k0 input; Te_values input; Lz_values input
function q_rad = fcn(Zeff, Te_tar, Te_omp, ne_omp, cz, k0, Te_values, Lz_values)

    % Usa interp1 per fare l'interpolazione
    Lz = @(Te) interp1(Te_values, Lz_values, Te, 'pchip', 'extrap');
    % Definisci l'integranda come una funzione anonima
    integrand = @(Te) Lz(Te) .* Te.^0.5 .* Zeff.^(-0.3);
    %disp(integrand)
    % Calcola l'integrale numerico tra Te_tar e Te_omp
    y = integral(integrand, Te_tar, Te_omp);
    %disp(y)
    %disp(cz)
    % q_rad = ne_omp*Te_omp*sqrt(2*max(0,cz)*k0*y);
    q_rad = ne_omp * Te_omp * sqrt(max(0, 2 * cz * k0 * y));
    %disp(q_rad)

end

== matlab function trasporto_impurezze/Trasporto particelle /MATLAB Function4 ==
  data: tau input; n_div input; tau1 input; n_div_dot output; n_tar input
function n_div_dot = fcn(tau, n_div, tau1, n_tar)
    % tau1 = 0.2;
    n_div_dot =  (n_tar-n_div)/tau1-(n_div)/tau;
end

== matlab function trasporto_impurezze/fourier/MATLAB Function2 ==
  data: alpha input; Tarea_dot output; Tarea input; Tomp input; Tdiv input; q_rad input
function Tarea_dot = fun(alpha, Tarea, Tomp, Tdiv,q_rad)
    Tarea_dot = (Tomp-Tarea)*alpha+(Tdiv-Tarea)*alpha-q_rad/3
end

== matlab function trasporto_impurezze/fourier/MATLAB Function3 ==
  data: alpha input; Tomp_dot output; Tarea input; Tomp input; P_cond input; q_rad input; rhocp input
function Tomp_dot = fun(alpha , Tarea,Tomp,P_cond,q_rad,rhocp)
    Tomp_dot = (Tarea-Tomp)*alpha+(P_cond)/(rhocp*0.014*3)-q_rad/3

end

== matlab function trasporto_impurezze/controllo T_core e calcolo P_cond/Dinamica - variazione temperatura/MATLAB Function2 ==
  data: cz input; ne input; P_imp output
function P_imp= fcn(cz, ne)
    P_imp = cz*ne^2*(10^-34)
end

== matlab function trasporto_impurezze/fourier/MATLAB Function1 ==
  data: alpha input; Tdiv_dot output; Tarea input; Tdiv input; Text input; gamma input; q_rad input
function Tdiv_dot = fun(alpha, Tarea, Tdiv, Text, gamma,q_rad)
  Tdiv_dot = (Tarea-Tdiv)*alpha+(Text-Tdiv)*gamma 
end

== matlab function trasporto_impurezze/controllo T_core e calcolo P_cond/Dinamica - variazione temperatura/Calcolo dE ==
  data: tau input; E input; dE output; Pnbi input; Pnbi0 input; P_brem input; P_imp input
function dE  = eqDiff(tau, E, Pnbi, Pnbi0, P_brem, P_imp)

    % delta = 1e-8; % Se E < soglia, => E = 0
    % k = 10;
    % stopSim = false;
    % 
    % if E < delta
    %     dE = 0;
    %     %stopSim = true; 
    % 
    % else
    dE = -(1/tau)*E + Pnbi+ Pnbi0 -P_brem -P_imp;
        
    % end
    % 
end

== matlab function trasporto_impurezze/controllo T_core e calcolo P_cond/Dinamica - variazione temperatura/MATLAB Function ==
  data: Zeff input; P_brem output; ni input; ne input; Te_core input
function P_brem = fcn(Zeff, ni, ne,Te_core)
    P_brem = (1.7*10^-38)*Zeff^2*ni*ne*sqrt(Te_core);
end

== matlab function trasporto_impurezze/MATLAB Function1 ==
  data: S input; n_core_dot output; n_omp input; n_core input; tau input
function n_core_dot = fcn(S, n_omp,n_core,tau)
    n_core_dot =  S+(n_omp-n_core)/tau;
    n_core_dot = 0;
end
